simulink model "octave_v2"  (R2018a)
settings: Solver=ode23t  StartTime=0.0  StopTime=0.1  MaxStep=1e-5  RelTol=1e-5
libraries: dspfdesign x2, simulink x1, simulink_extras x1, dspvision x1
settings Model: Creator=chris  LastModifiedBy=chris

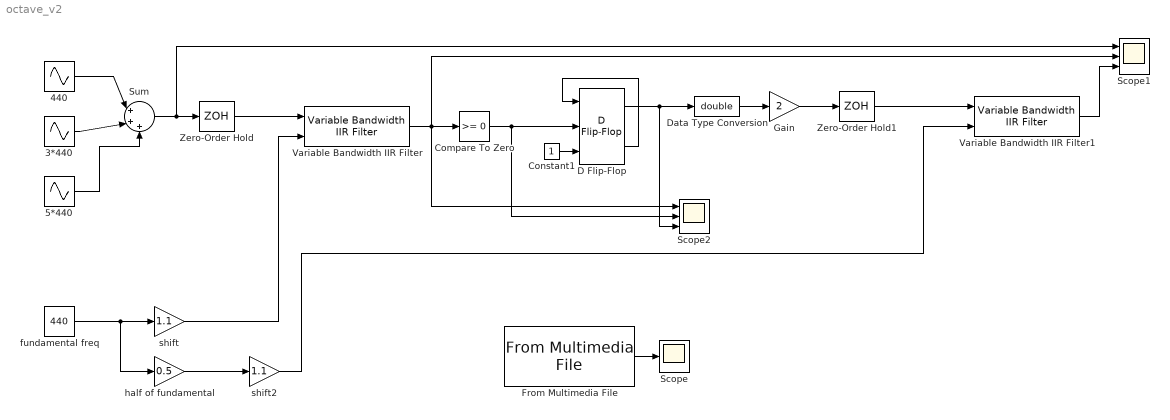
== system octave_v2 ==
  3*440 : Sin  Amplitude=0.5  Frequency=3*440*2*pi  SampleTime=0
  440 : Sin  Frequency=440*2*pi  SampleTime=0
  5*440 : Sin  Amplitude=0.1  Frequency=5*440*2*pi  SampleTime=0
  Compare To Zero : simulink/Logic and Bit Operations/Compare To Zero  relop=>=  OutDataTypeStr=boolean
  Constant1 : Constant
  D Flip-Flop : simulink_extras/Flip Flops/D Flip-Flop
      settings: SourceProductName=Simulink
  Data Type Conversion : DataTypeConversion  OutDataTypeStr=double
  From Multimedia File : dspvision/From Multimedia File  inputFilename=D:\Documents\programming\octave\simulink_v2\violin-C5.wav  loop=on  numPlays=inf  outputStreams=Audio only  videoDataType=single  audioDataType=double  inheritSampleTime=on  userDefinedSampleTime=1/30  noAudioOutput=off  isIntensityVideo=off  fourcc=RGB  colorVideoFormat=Separate color signals  outputEOF=off  dataOrg=Column-major  audioFrameSize=1024  computeAudioFrameSize=off  outSamplingMode=Sample based
      settings: SourceProductBaseCode=VP
  Gain : Gain  Gain=2
  Scope : Scope
  Scope1 : Scope  NumInputPorts=3
  Scope2 : Scope  NumInputPorts=3
  Sum : Sum  Inputs=|+++
  Variable Bandwidth IIR Filter : dspfdesign/Variable Bandwidth IIR Filter  FilterType=Lowpass  FilterOrder=8  PassbandFrequencyPort=on  PassbandFrequency=450  CenterFrequencyPort=off  CenterFrequency=44100/4  BandwidthPort=off  Bandwidth=7680  PassbandRipple=1  StopbandAttenuation=60  InheritSampleRate=off  SampleRate=44100  SimulateUsing=Code generation
      settings: SourceProductName=DSP System Toolbox  SourceProductBaseCode=DS
  Variable Bandwidth IIR Filter1 : dspfdesign/Variable Bandwidth IIR Filter  FilterType=Lowpass  FilterOrder=8  PassbandFrequencyPort=on  PassbandFrequency=450  CenterFrequencyPort=off  CenterFrequency=44100/4  BandwidthPort=off  Bandwidth=7680  PassbandRipple=1  StopbandAttenuation=60  InheritSampleRate=off  SampleRate=44100  SimulateUsing=Code generation
      settings: SourceProductName=DSP System Toolbox  SourceProductBaseCode=DS
  Zero-Order Hold : ZeroOrderHold  SampleTime=-1
  Zero-Order Hold1 : ZeroOrderHold  SampleTime=-1
  fundamental freq : Constant  Value=440
  half of fundamental : Gain  Gain=0.5
  shift : Gain  Gain=1.1
  shift2 : Gain  Gain=1.1
  wires:
  440/1 -> Sum/1
  3*440/1 -> Sum/2
  Variable Bandwidth IIR Filter/1 -> Scope1/2, Scope2/1, Compare To Zero/1
  Zero-Order Hold/1 -> Variable Bandwidth IIR Filter/1
  5*440/1 -> Sum/3
  shift/1 -> Variable Bandwidth IIR Filter/2
  Compare To Zero/1 -> Scope2/2, D Flip-Flop/2
  Constant1/1 -> D Flip-Flop/3
  D Flip-Flop/2 -> D Flip-Flop/1
  D Flip-Flop/1 -> Data Type Conversion/1, Scope2/3
  Data Type Conversion/1 -> Gain/1
  Gain/1 -> Zero-Order Hold1/1
  Variable Bandwidth IIR Filter1/1 -> Scope1/3
  shift2/1 -> Variable Bandwidth IIR Filter1/2
  Zero-Order Hold1/1 -> Variable Bandwidth IIR Filter1/1
  fundamental freq/1 -> half of fundamental/1, shift/1
  half of fundamental/1 -> shift2/1
  Sum/1 -> Scope1/1, Zero-Order Hold/1
  From Multimedia File/1 -> Scope/1
